simulink model "demo_lab5"  (R2023a)
settings: Solver=VariableStepAuto  StartTime=0.0  StopTime=5  RelTol=1e-3
libraries: simulink x3
settings Model: Creator=mhb  LastModifiedBy=Dylan
settings OptimizationCC: ReuseModelBlockBuffer=off

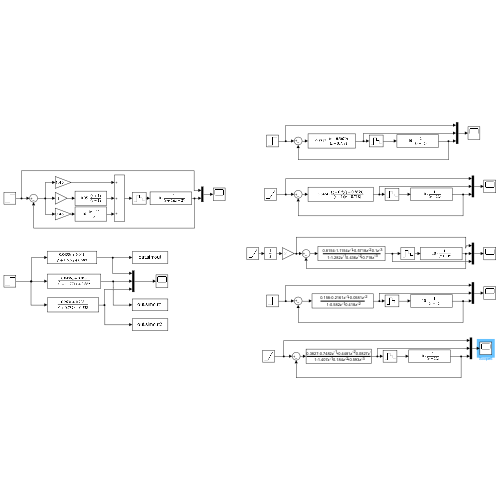
[thumbnail: Simulink's stored preview of the top-level diagram]
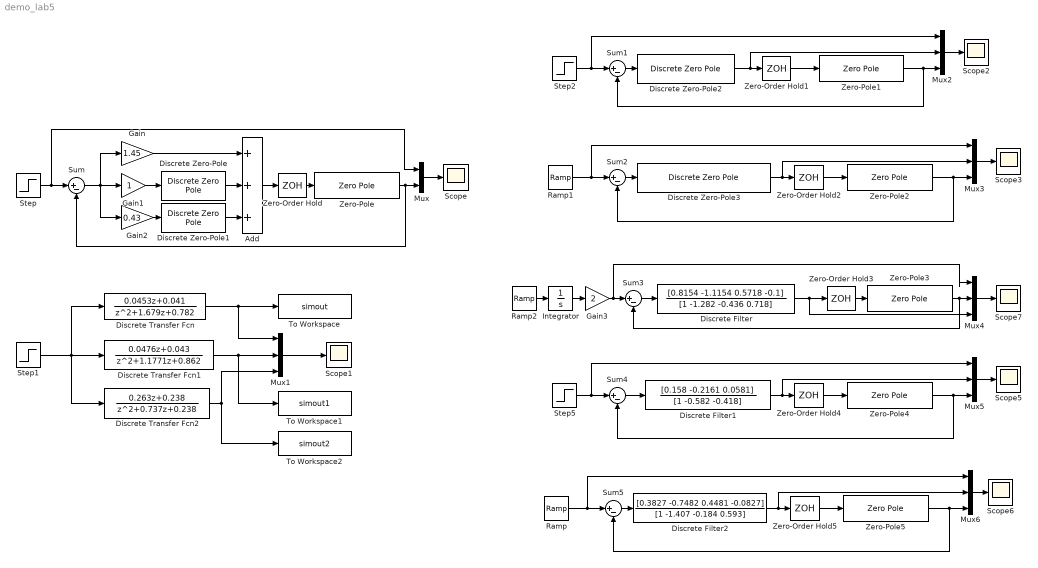
== system demo_lab5 ==
  Add : Sum  Inputs=+++
  Discrete Transfer Fcn : DiscreteTransferFcn  Numerator=[0.0453 0.041]  Denominator=[1 1.679 0.782]  SampleTime=0.1
  Discrete Transfer Fcn1 : DiscreteTransferFcn  Numerator=[0.0476 0.043]  Denominator=[1 1.1771 0.862]  SampleTime=0.1
  Discrete Transfer Fcn2 : DiscreteTransferFcn  Numerator=[0.263 0.238]  Denominator=[1 0.737 0.238]  SampleTime=0.1
  Discrete Zero-Pole : DiscreteZeroPole  Zeros=[-1]  Poles=[1]  Gain=0.05  SampleTime=0.1
  Discrete Zero-Pole1 : DiscreteZeroPole  Poles=[0]  Gain=10  SampleTime=0.1
  Discrete Zero-Pole2 : DiscreteZeroPole  Zeros=[0.3679]  Poles=[0.718]  Gain=0.2717
  Discrete Zero-Pole3 : DiscreteZeroPole  Zeros=[0.5 0.3679]  Poles=[1 -0.718]  Gain=0.5434
  Discrete Filter : DiscreteFilter  Numerator=[0.8154 -1.1154 0.5718 -0.1]  Denominator=[1 -1.282 -0.436 0.718]  SampleTime=1
  Discrete Filter1 : DiscreteFilter  Numerator=[0.158 -0.2161 0.0581]  Denominator=[1 -0.582 -0.418]  SampleTime=1
  Discrete Filter2 : DiscreteFilter  Numerator=[0.3827 -0.7482 0.4481 -0.0827]  Denominator=[1 -1.407 -0.184 0.593]  SampleTime=1
  Gain : Gain  Gain=1.45
  Gain1 : Gain
  Gain2 : Gain  Gain=0.43
  Gain3 : Gain  Gain=2
  Integrator : Integrator
  Mux : Mux  Inputs=2
  Mux{1..6} (6 alike) : Mux  Inputs=3
  Ramp : simulink/Sources/Ramp  slope=1  start=0  InitialOutput=0
  Ramp1 : simulink/Sources/Ramp  slope=1  start=0  InitialOutput=0
  Ramp2 : simulink/Sources/Ramp  slope=1  start=0  InitialOutput=0
  Scope{,1..3,5..7} (7 alike) : Scope
  Step{,1..2,5} (4 alike) : Step  Time=0  SampleTime=0
  Sum{,1..5} (6 alike) : Sum  Inputs=|+-
  To Workspace : ToWorkspace  VariableName=simout  SaveFormat=Timeseries  SampleTime=-1
  To Workspace1 : ToWorkspace  VariableName=simout1  SaveFormat=Timeseries  SampleTime=-1
  To Workspace2 : ToWorkspace  VariableName=simout2  SaveFormat=Timeseries  SampleTime=-1
  Zero-Order Hold{,1..5} (6 alike) : ZeroOrderHold  SampleTime=-1
  Zero-Pole : ZeroPole  Zeros=[ ]  Poles=[-1 -2]  Gain=10
  Zero-Pole{1..5} (5 alike) : ZeroPole  Zeros=[ ]  Poles=[-1 0]  Gain=10
  wires:
  Add/1 -> Zero-Order Hold/1
  Zero-Order Hold/1 -> Zero-Pole/1
  Mux/1 -> Scope/1
  Zero-Pole/1 -> Mux/2, Sum/2
  Step/1 -> Mux/1, Sum/1
  Sum/1 -> Gain2/1, Gain/1, Gain1/1
  Gain1/1 -> Discrete Zero-Pole/1
  Discrete Zero-Pole/1 -> Add/2
  Discrete Zero-Pole1/1 -> Add/3
  Gain/1 -> Add/1
  Gain2/1 -> Discrete Zero-Pole1/1
  Mux1/1 -> Scope1/1
  Discrete Transfer Fcn2/1 -> Mux1/3, To Workspace2/1
  Discrete Transfer Fcn1/1 -> To Workspace1/1, Mux1/2
  Discrete Transfer Fcn/1 -> Mux1/1, To Workspace/1
  Step1/1 -> Discrete Transfer Fcn/1, Discrete Transfer Fcn1/1, Discrete Transfer Fcn2/1
  Step2/1 -> Sum1/1, Mux2/1
  Zero-Order Hold1/1 -> Zero-Pole1/1
  Zero-Pole1/1 -> Sum1/2, Mux2/3
  Mux2/1 -> Scope2/1
  Discrete Zero-Pole2/1 -> Mux2/2, Zero-Order Hold1/1
  Sum1/1 -> Discrete Zero-Pole2/1
  Sum2/1 -> Discrete Zero-Pole3/1
  Discrete Zero-Pole3/1 -> Mux3/2, Zero-Order Hold2/1
  Mux3/1 -> Scope3/1
  Zero-Pole2/1 -> Mux3/3, Sum2/2
  Zero-Order Hold2/1 -> Zero-Pole2/1
  Ramp1/1 -> Mux3/1, Sum2/1
  Sum3/1 -> Discrete Filter/1
  Zero-Pole3/1 -> Mux4/2, Sum3/2
  Discrete Filter/1 -> Mux4/3, Zero-Order Hold3/1
  Zero-Order Hold3/1 -> Zero-Pole3/1
  Integrator/1 -> Gain3/1
  Step5/1 -> Sum4/1, Mux5/1
  Zero-Order Hold4/1 -> Zero-Pole4/1
  Zero-Pole4/1 -> Sum4/2, Mux5/3
  Mux5/1 -> Scope5/1
  Discrete Filter1/1 -> Zero-Order Hold4/1, Mux5/2
  Sum4/1 -> Discrete Filter1/1
  Sum5/1 -> Discrete Filter2/1
  Discrete Filter2/1 -> Mux6/2, Zero-Order Hold5/1
  Mux6/1 -> Scope6/1
  Zero-Pole5/1 -> Mux6/3, Sum5/2
  Zero-Order Hold5/1 -> Zero-Pole5/1
  Ramp/1 -> Mux6/1, Sum5/1
  Gain3/1 -> Mux4/1, Sum3/1
  Mux4/1 -> Scope7/1
  Ramp2/1 -> Integrator/1
